simulink model "Motorcycle_stability"  (Simulink 6.5)
settings: Solver=ode15s  StartTime=0.0  StopTime=2  RelTol=1e-6
values from neighbouring files (symbols this model uses):
  Arel = A(states, states)    [Bicycle_StateSpaceController_LeanSteer_RiderLean.m]    (also in ControllerParameterDesign.m; EV_SL2001.m; LQR_Controller.m; LeanControl.m)
  As = Arel - Brel*F    [ControllerParameterDesign.m]
  Brel = B(states,:)    [Bicycle_StateSpaceController_LeanSteer_RiderLean.m]    (also in ControllerParameterDesign.m; EV_SL2001.m; LQR_Controller.m; LeanControl.m)
  Crel = eye(2)    [ControllerParameterDesign.m]    (also in StateSpaceController_LeanLateral.m = C(:,states))
  F = place2(Arel, Brel, poles)    [Bicycle_StateSpaceController_LeanSteer_RiderLean.m]    (also in ControllerParameterDesign.m = place(Arel, Brel, [p1, p2]); LQR_Controller.m = lqr(Arel, Brel, Q, R); LeanControl.m = place(Arel, Brel, [p1, p2]); StateSpaceController_LeanLateral.m = place(Arel, Brel, [p1, p2, p3, p4]))
  xs = [delta, 0, phi, 0]    [ControllerParameterDesign.m]
settings Model: Creator=Thomas  LastModifiedBy=Thomas

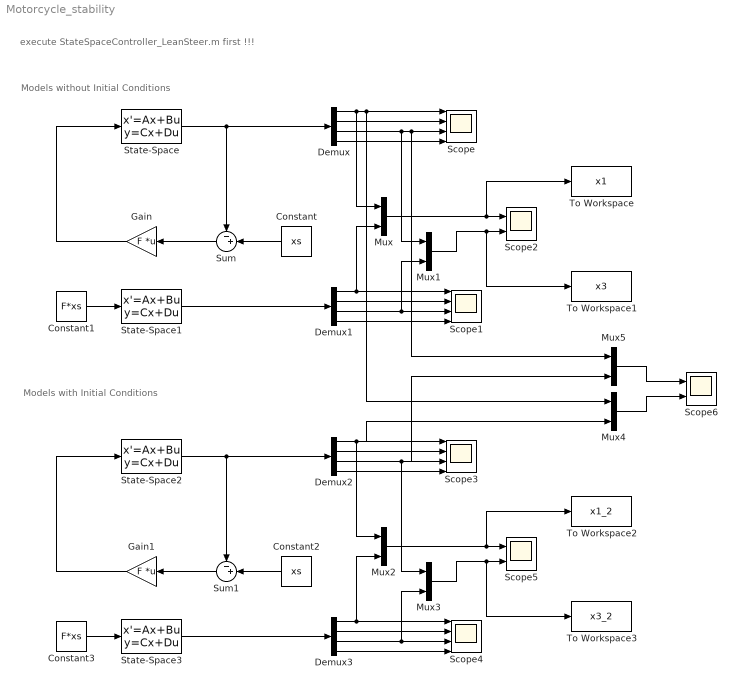
== system Motorcycle_stability ==
  note: execute StateSpaceController_LeanSteer.m first !!!
  note: Models without Initial Conditions
  note: Models with Initial Conditions
  Constant : Constant  Orientation=left  Value=xs  OutDataType=sfix(16)  ConRadixGroup=Use specified scaling  OutScaling=2^0  SampleTime=inf  FramePeriod=inf
  Constant1 : Constant  Value=F*xs  OutDataType=sfix(16)  ConRadixGroup=Use specified scaling  OutScaling=2^0  SampleTime=inf  FramePeriod=inf
  Constant2 : Constant  Orientation=left  Value=xs  OutDataType=sfix(16)  ConRadixGroup=Use specified scaling  OutScaling=2^0  SampleTime=inf  FramePeriod=inf
  Constant3 : Constant  Value=F*xs  OutDataType=sfix(16)  ConRadixGroup=Use specified scaling  OutScaling=2^0  SampleTime=inf  FramePeriod=inf
  Demux{,1..3} (4 alike) : Demux
  Gain : Gain  Orientation=left  Gain=F  Multiplication=Matrix(K*u)
  Gain1 : Gain  Orientation=left  Gain=F  Multiplication=Matrix(K*u)
  Mux{,1..5} (6 alike) : Mux  Inputs=2
  Scope{,1,3..4} (4 alike) : Scope  NumInputPorts=4
      Scope settings: TimeRange=0.8  YMin=0.396088~-5~-5~-5  YMax=4.39609~5~5~5
      Scope1 settings: TimeRange=0.8  YMin=0.396088~-5~-5~-5  YMax=4.39609~5~5~5
      Scope3 settings: TimeRange=2  YMin=-0.02~-1~0~0  YMax=0.03999999999999999~1~0.4~1.5  SaveName=ScopeData3
      Scope4 settings: TimeRange=0.8  YMin=0.396088~-5~-5~-5  YMax=4.39609~5~5~5  SaveName=ScopeData4
  Scope2 : Scope  NumInputPorts=2
      settings: TimeRange=2  YMin=-0.02~0  YMax=0.03999999999999999~0.35  SaveName=ScopeData2
  Scope5 : Scope  NumInputPorts=2
      settings: TimeRange=2  YMin=-0.015~0.05  YMax=0.025~0.3  SaveName=ScopeData5
  Scope6 : Scope  NumInputPorts=2
      settings: TimeRange=2  YMin=0~-0.02  YMax=0.35~0.03999999999999999  SaveName=ScopeData6
  State-Space : StateSpace  A=Arel  B=Brel  C=Crel  D=[ 0 0 0 0 ]'
  State-Space1 : StateSpace  A=As  B=Brel  C=Crel  D=[ 0 0 0 0 ]'
  State-Space2 : StateSpace  A=Arel  B=Brel  C=Crel  D=[ 0 0 0 0 ]'  X0=[0 0 5*pi/180 0]'
  State-Space3 : StateSpace  A=As  B=Brel  C=Crel  D=[ 0 0 0 0 ]'  X0=[0 0 5*pi/180 0]'
  Sum : Sum  Orientation=left  Inputs=-+|
  Sum1 : Sum  Orientation=left  Inputs=-+|
  To Workspace : ToWorkspace  VariableName=x1  SampleTime=-1  SaveFormat=Structure With Time
  To Workspace1 : ToWorkspace  VariableName=x3  SampleTime=-1  SaveFormat=Structure With Time
  To Workspace2 : ToWorkspace  VariableName=x1_2  SampleTime=-1  SaveFormat=Structure With Time
  To Workspace3 : ToWorkspace  VariableName=x3_2  SampleTime=-1  SaveFormat=Structure With Time
  wires:
  Constant/1 -> Sum/2
  Gain/1 -> State-Space/1
  Sum/1 -> Gain/1
  State-Space/1 -> Demux/1, Sum/1
  Demux/1 -> Mux/1, Scope/1, Mux4/1
  Demux/2 -> Scope/2
  Demux/3 -> Mux1/1, Scope/3, Mux5/1
  Demux/4 -> Scope/4
  State-Space1/1 -> Demux1/1
  Demux1/1 -> Scope1/1, Mux/2
  Demux1/2 -> Scope1/2
  Demux1/3 -> Scope1/3, Mux1/2
  Demux1/4 -> Scope1/4
  Constant1/1 -> State-Space1/1
  Mux/1 -> Scope2/1, To Workspace/1
  Mux1/1 -> Scope2/2, To Workspace1/1
  Constant2/1 -> Sum1/2
  Gain1/1 -> State-Space2/1
  Sum1/1 -> Gain1/1
  State-Space2/1 -> Demux2/1, Sum1/1
  Demux2/1 -> Scope3/1, Mux2/1, Mux4/2
  Demux2/2 -> Scope3/2
  Demux2/3 -> Scope3/3, Mux3/1, Mux5/2
  Demux2/4 -> Scope3/4
  State-Space3/1 -> Demux3/1
  Demux3/1 -> Scope4/1, Mux2/2
  Demux3/2 -> Scope4/2
  Demux3/3 -> Scope4/3, Mux3/2
  Demux3/4 -> Scope4/4
  Constant3/1 -> State-Space3/1
  Mux2/1 -> Scope5/1, To Workspace2/1
  Mux3/1 -> Scope5/2, To Workspace3/1
  Mux5/1 -> Scope6/1
  Mux4/1 -> Scope6/2
